simulink model "Lab4"  (R2017b)
settings: Solver=FixedStepDiscrete  StartTime=0.0  StopTime=inf  RelTol=1e-3  EnableMultiTasking=on
undefined symbols (not defined in the file or in its folder): Green, led0
libraries: simulink x1, embdlinuxlib x1
settings Model: SimulationMode=external  Creator=tommy  LastModifiedBy=bjorn
settings SolverCC: PositivePriorityOrder=on
settings OptimizationCC: LifeSpan=1  MaxStackSize=64
settings DebuggingCC: SFUnexpectedBacktrackingDiag=warning  SFNoUnconditionalDefaultTransitionDiag=warning  SFExecutionAtInitializationDiag=none
settings HardwareCC: ProdBitPerPointer=32  ProdBitPerSizeT=32  ProdBitPerPtrDiffT=32  ProdLargestAtomicInteger=Long  ProdLargestAtomicFloat=Double  ProdWordSize=32  ProdHWDeviceType=ARM Compatible->ARM Cortex
settings SFSimCC: MATLABDynamicMemAlloc=off
settings RTWCC: SystemTargetFile=ert.tlc  HardwareBoard=Raspberry Pi  TLCOptions=-aInlineSetEventsForThisBaseRateFcn=TLC_FALSE -aSuppressMultiTaskScheduler=TLC_FALSE -aRateBasedStepFcn=0  TemplateMakefile=ert_default_tmf  Toolchain=GNU GCC Raspberry Pi
settings CodeAppCC: ForceParamTrailComments=on  IgnoreCustomStorageClasses=off  OperatorAnnotations=on  SimulinkDataObjDesc=on  SFDataObjDesc=on  MATLABFcnDesc=on  InsertBlockDesc=on  StateflowObjectComments=on  MATLABSourceComments=on
settings ERTTargetCC: MultiwordLength=2048  SupportVariableSizeSignals=on
settings ConfigComp: CovMetricSettings=dw  CovHtmlReporting=on  CovSaveCumulativeToWorkspaceVar=on  CovSaveSingleToWorkspaceVar=on  CovExternalEMLEnable=off

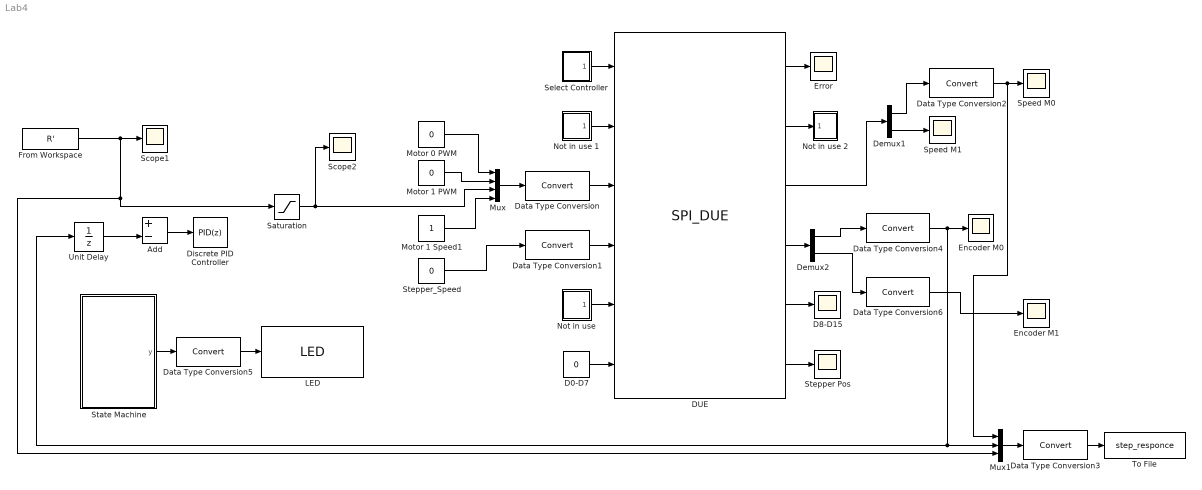
== system Lab4 ==
  Add : Sum  Inputs=+-
  D0-D7 : Constant  Value=0  OutDataTypeStr=uint8
  D8-D15 : Scope
  DUE : S-Function  InitFcn=try, set_param(gcb,'FunctionName','SPI_DUE'), end  FunctionName=SPI_DUE  Parameters=uint8(1),uint32(4000000)  SFunctionModules=SPI_DUE_wrapper  SFunctionDeploymentMode=off  EnableBusSupport=off  mask(S-Function Builder){}
      mask help: Simulink:masks:SFunctionBuilder_MD
      mask init:
      | val = [[.9  0.75 0.75 1 1 .9 .9 1]',[1 1 0.75 0.75 .9 .9 1 .9]'];try , sys = get_param(gcb,'SfunBuilderFcnName');if isempty(sys), sys = get_param(gcb,'FunctionName'); end,catch, sys = get_param(gcb,'FunctionName'); end
      settings: CopyFcn=set_param(gcbh,'LinkStatus','none')  PreSaveFcn=try, set_param(gcb,'FunctionName','SPI_DUE'), end  OpenFcn=sfunctionwizard(gcbh)
      mask Display: plot(val(:,1),val(:,2)),disp(sys), port_label('input',1,'Select'), port_label('input',2,'Sample_Time'), port_label('input',3,'Set_Speed_DC'), port_label('input',4,'Set_Speed_Stepper'), port_label('input',5,'Controllers'), port_label('input',6,'Set_Digital'), port_label('output',1,'Status'), port_label('output',2,'Current'), port_label('output',3,'Motor_Speed'), port_label('output',4,'Motor_Encoder'), port_label('output',5,'Read_Digital'), port_label('output',6,'Stepper_Pos')
  Data Type Conversion{,1..6} (7 alike) : DataTypeConversion
  Demux1 : Demux  Outputs=2
  Demux2 : Demux  Outputs=2
  Discrete PID Controller : simulink/Continuous/PID Controller  Controller=PID  TimeDomain=Discrete-time  SampleTime=-1  IntegratorMethod=Forward Euler  FilterMethod=Forward Euler  Form=Parallel  UseFilter=on  ControllerParametersSource=internal  P=0.1  I=0.02  D=0  N=1000  InitialConditionSource=internal  InitialConditionForIntegrator=0  InitialConditionForFilter=0  ExternalReset=none  LimitOutput=off  UpperSaturationLimit=inf  LowerSaturationLimit=-inf  LinearizeAsGain=off  AntiWindupMode=none  Kb=1  TrackingMode=off  Kt=1  PParamMin=[]  PParamMax=[]  IParamMin=[]  IParamMax=[]  DParamMin=[]  DParamMax=[]  NParamMin=[]  NParamMax=[]  KbParamMin=[]  KbParamMax=[]  KtParamMin=[]  KtParamMax=[]  POutMin=[]  POutMax=[]  IOutMin=[]  IOutMax=[]  DOutMin=[]  DOutMax=[]  NOutMin=[]  NOutMax=[]  KbOutMin=[]  KbOutMax=[]  KtOutMin=[]  KtOutMax=[]  IntegratorOutMin=[]  IntegratorOutMax=[]  FilterOutMin=[]  FilterOutMax=[]  SumOutMin=[]  SumOutMax=[]  SumI1OutMin=[]  SumI1OutMax=[]  SumI2OutMin=[]  SumI2OutMax=[]  SumI3OutMin=[]  SumI3OutMax=[]  SumDOutMin=[]  SumDOutMax=[]  SaturationOutMin=[]  SaturationOutMax=[]  IntegratorContinuousStateAttributes=''  IntegratorStateMustResolveToSignalObject=off  IntegratorRTWStateStorageClass=Auto  FilterContinuousStateAttributes=''  FilterStateMustResolveToSignalObject=off  FilterRTWStateStorageClass=Auto  DifferentiatorICPrevScaledInput=0  DifferentiatorOutMin=[]  DifferentiatorOutMax=[]  InitialConditionSetting=State (most efficient)  FilterDiffOutCoefMin=[]  FilterDiffOutCoefMax=[]  SumDenOutMin=[]  SumDenOutMax=[]  SumNumOutMin=[]  SumNumOutMax=[]  ReciprocalOutMin=[]  ReciprocalOutMax=[]  DivideOutMin=[]  DivideOutMax=[]  TunerSelectOption=Transfer Function Based (PID Tuner App)
  Encoder M0 : Scope
  Encoder M1 : Scope
  Error : Scope
  From Workspace : FromWorkspace  VariableName=R'  SampleTime=0.01
  LED : embdlinuxlib/LED  board=Model B+  led=led0 (Green)  blockPlatform=Raspberry Pi
      settings: SourceProductName=Simulink Support Package for Raspberry Pi Hardware  SourceProductBaseCode=RASPPI
  Motor 0 PWM : Constant  Value=0
  Motor 1 PWM : Constant  Value=0
  Motor 1 Speed1 : Constant
  Mux : Mux
  Mux1 : Mux  Inputs=3
  Not in use : Subsystem
  Not in use 1 : Subsystem
  Not in use 2 : Subsystem
  Saturation : Saturate  UpperLimit=1000  LowerLimit=-2000
  Scope1 : Scope
  Scope2 : Scope
  Select Controller : Subsystem
  Speed M0 : Scope
  Speed M1 : Scope
  State Machine : Stateflow chart  TreatAsAtomicUnit=on
  Stepper Pos : Scope
  Stepper_Speed : Constant  Value=0
  To File : ToFile  Filename=step_responce
  Unit Delay : UnitDelay  SampleTime=-1
  wires:
  Mux/1 -> Data Type Conversion/1
  DUE/1 -> Error/1
  Data Type Conversion/1 -> DUE/3
  DUE/5 -> D8-D15/1
  DUE/4 -> Demux2/1
  Not in use 1/1(Out1) -> DUE/2
  Select Controller/1(Out1) -> DUE/1
  DUE/2 -> Not in use 2/1(In1)
  DUE/3 -> Demux1/1
  Not in use/1(Out1) -> DUE/5
  Data Type Conversion3/1 -> To File/1
  Motor 1 PWM/1 -> Mux/2
  Mux1/1 -> Data Type Conversion3/1
  Data Type Conversion4/1 -> Mux1/2, Unit Delay/1, Encoder M0/1
  Demux2/1 -> Data Type Conversion4/1
  DUE/6 -> Stepper Pos/1
  D0-D7/1 -> DUE/6
  Data Type Conversion1/1 -> DUE/4
  Demux1/2 -> Speed M1/1
  Demux1/1 -> Data Type Conversion2/1
  Data Type Conversion2/1 -> Mux1/1, Speed M0/1
  Data Type Conversion5/1 -> LED/1
  State Machine/1(y) -> Data Type Conversion5/1
  Stepper_Speed/1 -> Data Type Conversion1/1
  Saturation/1 -> Scope2/1, Mux/3
  From Workspace/1 -> Saturation/1, Mux1/3, Scope1/1
  Motor 0 PWM/1 -> Mux/1
  Motor 1 Speed1/1 -> Mux/4
  Demux2/2 -> Data Type Conversion6/1
  Data Type Conversion6/1 -> Encoder M1/1
  Unit Delay/1 -> Add/2
  Add/1 -> Discrete PID Controller/1

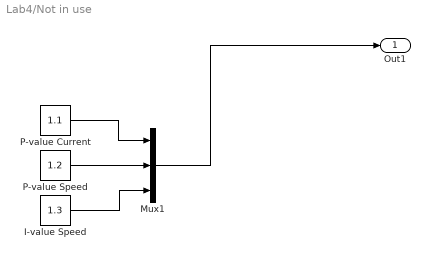
== system Lab4/Not in use ==
  I-value Speed : Constant  Value=1.3  OutDataTypeStr=single
  Mux1 : Mux  Inputs=3
  P-value Current : Constant  Value=1.1  OutDataTypeStr=single
  P-value Speed : Constant  Value=1.2  OutDataTypeStr=single
  Out1 : Outport
  wires:
  Mux1/1 -> Out1/1
  P-value Current/1 -> Mux1/1
  I-value Speed/1 -> Mux1/3
  P-value Speed/1 -> Mux1/2

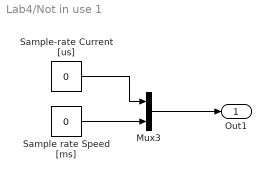
== system Lab4/Not in use 1 ==
  Mux3 : Mux  Inputs=2
  Sample rate Speed [ms] : Constant  Value=0  OutDataTypeStr=uint16
  Sample-rate Current [us] : Constant  Value=0  OutDataTypeStr=uint16
  Out1 : Outport
  wires:
  Sample-rate Current [us]/1 -> Mux3/1
  Mux3/1 -> Out1/1
  Sample rate Speed [ms]/1 -> Mux3/2

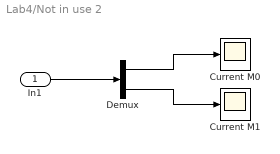
== system Lab4/Not in use 2 ==
  In1 : Inport
  Current M0 : Scope
  Current M1 : Scope
  Demux : Demux  Outputs=2
  wires:
  In1/1 -> Demux/1
  Demux/2 -> Current M1/1
  Demux/1 -> Current M0/1

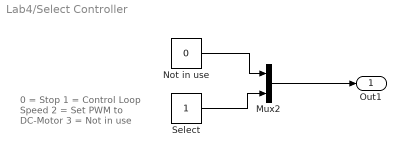
== system Lab4/Select Controller ==
  note: 0 = Stop
      | 1 = Control Loop Speed
      | 2 = Set PWM to DC-Motor
      | 3 = Not in use
  Mux2 : Mux  Inputs=2
  Not in use : Constant  Value=0  OutDataTypeStr=uint8
  Select : Constant  OutDataTypeStr=uint8
  Out1 : Outport
  wires:
  Select/1 -> Mux2/2
  Not in use/1 -> Mux2/1
  Mux2/1 -> Out1/1

== stateflow chart Lab4/State Machine ==
  state Led_off
    entry:
    y=0;
    Counter = 0;
    during:
    Counter = Counter + 1;
  state Led_on
    entry:
    y=1;
  Led_off -> Led_on : [Counter > 10]
  (default) -> Led_off
  Led_on -> Led_off : after(2,sec)
  data: y output; Counter local
